simulink model "serialCom"  (R2023a)
settings: Solver=VariableStepAuto  StartTime=0.0  StopTime=inf  RelTol=1e-3
model workspace (MAT data in the model file):
  R = 0
undefined symbols (not defined in the file): LF
libraries: instrumentseriallib x2
settings Model: Creator=zoro  LastModifiedBy=zoro

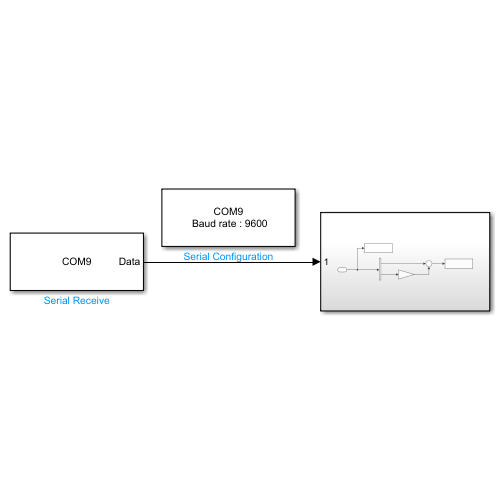
[thumbnail: Simulink's stored preview of the top-level diagram]
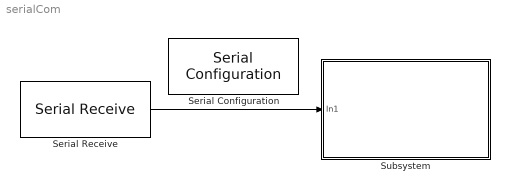
== system serialCom ==
  Serial Configuration : instrumentseriallib/Serial Configuration  Priority=-200000  PortSel=COM9  Port=COM9  ComPort=COM9  BaudRate=9600  DataBits=8  Parity=none  StopBits=1  ByteOrder=little-endian  FlowControl=none  Timeout=10  SimulateUsing=Interpreted execution  BlockInModel=on  aMode=1
  Serial Receive : instrumentseriallib/Serial Receive  Priority=1  PortSel=COM9  Port=COM9  ComPort=COM9  DataType=uint8  SaveDataType=uint8  ToggleHeader=on  Header=R  ToggleTerminator=on  Terminator=LF ('\n')  CustomTerminator=[]  InputFormat=Column major  ToggleDataSize=on  DataSize=1  EnableBlockingMode=on  ActionDataUnavailable=Output last received value  ActionWhenDataUnavailable=Output last received value  CustomValue=0  SampleTime=0.01  SimulateUsing=Interpreted execution  BlockInModel=on  aMode=1
  Subsystem : Subsystem
  wires:
  Serial Receive/1 -> Subsystem/1(In1)

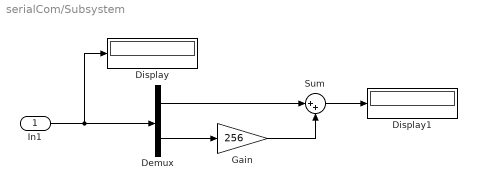
== system serialCom/Subsystem ==
  In1 : Inport
  Demux : Demux  Outputs=2
  Display : Display
  Display1 : Display
  Gain : Gain  Gain=256
  Sum : Sum  Inputs=|++
  wires:
  Sum/1 -> Display1/1
  Demux/1 -> Sum/1
  Gain/1 -> Sum/2
  In1/1 -> Display/1, Demux/1
  Demux/2 -> Gain/1
